simulink model "VIPR557StEnCtrl"  (R2018b)
settings: Solver=FixedStepDiscrete  StartTime=0.0  StopTime=10.0  FixedStep=0.01  RelTol=1e-3
undefined symbols (not defined in the file or in its folder): data, KeSMSw4SSecRwLtStLgrstUpwdDnwdOpenPos1_Val, PassStBkReclnEn_Clear, PassStBkReclnEn_Set, PassStFwdBkwdEn_Clear, PassStFwdBkwdEn_Set, SecRwRtStBkReclnEn_Clear, SecRwRtStBkReclnEn_Set, SecRwRtStFwdBkwdEn_Clear, SecRwRtStFwdBkwdEn_Set, SecRwRtStLgrstInwdOtwdEn_Clear, SecRwRtStLgrstInwdOtwdEn_Set, SecRwRtStLgrstUpwdDnwdEn_Clear, SecRwRtStLgrstUpwdDnwdEn_Set, ThdRwLtStBkReclnEn_Clear, ThdRwLtStBkReclnEn_Set, ThdRwLtStFwdBkwdEn_Clear, ThdRwLtStFwdBkwdEn_Set, ThdRwRtStBkReclnEn_Clear, ThdRwRtStBkReclnEn_Set, ThdRwRtStFwdBkwdEn_Clear, ThdRwRtStFwdBkwdEn_Set, ZeroREn_Clear, ZeroREn_Set
libraries: simulink x1
settings Model: Creator=sn2xws  LastModifiedBy=sn2xws
settings Model: ModifiedHistory=|
  | 2024.7.3 V3.0.0 557模式流程V1.9
  | 2024.8.16 V3.0.1  目标位置改为立即读取
  | 2024.8.22 V3.0.2 增加FirstTrig参数，智享目标位置计算改为只计算一次
  | 2024.8.30 V3.0.3 修复第一次无法调用问题
  | 2024.10.28 V3.0.4 6s版本不动三左
  | 2024.11.5 V3.0.5 6s版本不动三左更改逻辑错误，stateflow改为！7s
  | 2024.12.11 v3.0.6 CR953605
  | 2025.03.28 V3.0.7 CR1010402
  | 2025.04.07 V3.0.8 CR1010402 靠背位置无效。前后靠背电机都不动
  | 2025.6.25 V3.13.0 bug1068643 腿托流程偶发提前问题修复
  | 25.7.31 V3.13.1 CR 1100249
  | 25.9.12 V3.16.0 优化副驾占座后的动作（不恢复动作）
settings DataIOCC: SaveFormat=StructureWithTime
settings OptimizationCC: DefaultParameterBehavior=Inlined  EnhancedBackFolding=on  PassReuseOutputArgsAs=Individual arguments  ZeroExternalMemoryAtStartup=off  ZeroInternalMemoryAtStartup=off  OptimizeBlockOrder=speed  DifferentSizesBufferReuse=on  OptimizationCustomize=off
settings DebuggingCC: ParameterTunabilityLossMsg=error
settings SFSimCC: MATLABDynamicMemAlloc=off
settings RTWCC: SystemTargetFile=autosar.tlc  GenCodeOnly=on  TemplateMakefile=ert_default_tmf  Description=AUTOSAR  GenerateReport=on  IncludeHyperlinkInReport=on  LaunchReport=on  GenerateTraceInfo=on  GenerateTraceReport=on  GenerateTraceReportSl=on  GenerateTraceReportSf=on  GenerateTraceReportEml=on
settings CodeAppCC: ForceParamTrailComments=on  IgnoreCustomStorageClasses=off  OperatorAnnotations=on  SimulinkDataObjDesc=on  SFDataObjDesc=on  InsertBlockDesc=on
settings STFCustomTargetCC: TargetLangStandard=C99 (ISO)  MultiwordLength=256  ParMdlRefBuildCompliant=on  CompOptLevelCompliant=on  IncludeMdlTerminateFcn=off  CombineOutputUpdateFcns=on  SuppressErrorStatus=on  ERTCustomFileBanners=on  SupportNonFinite=off  SupportComplex=off  SupportContinuousTime=off  SupportNonInlinedSFcns=off  RemoveResetFunc=on  MATLABClassNameForMDSCustomization=Simulink.SoftwareTarget.ERTCustomization  AutosarCompliant=on  UseToolchainInfoCompliant=on  LookupTableObjectStructAxisOrder=2,1,3,4,...  LUTObjectStructOrderEvenSpacing=Size,Table,Breakpoints  SystemTargetFile=autosar.tlc
settings ERTTargetCC: TargetLangStandard=C99 (ISO)  ConcurrentExecutionCompliant=off  IncludeMdlTerminateFcn=off  SuppressErrorStatus=on  SupportNonFinite=off  SupportComplex=off  ModelStepFunctionPrototypeControlCompliant=off  CPPClassGenCompliant=off  AutosarCompliant=on  LookupTableObjectStructAxisOrder=2,1,3,4,...  LUTObjectStructOrderEvenSpacing=Size,Table,Breakpoints  InlinedParameterPlacement=NonHierarchical  ERTCustomFileTemplate=example_file_process.tlc  ERTFilePackagingFormat=Compact

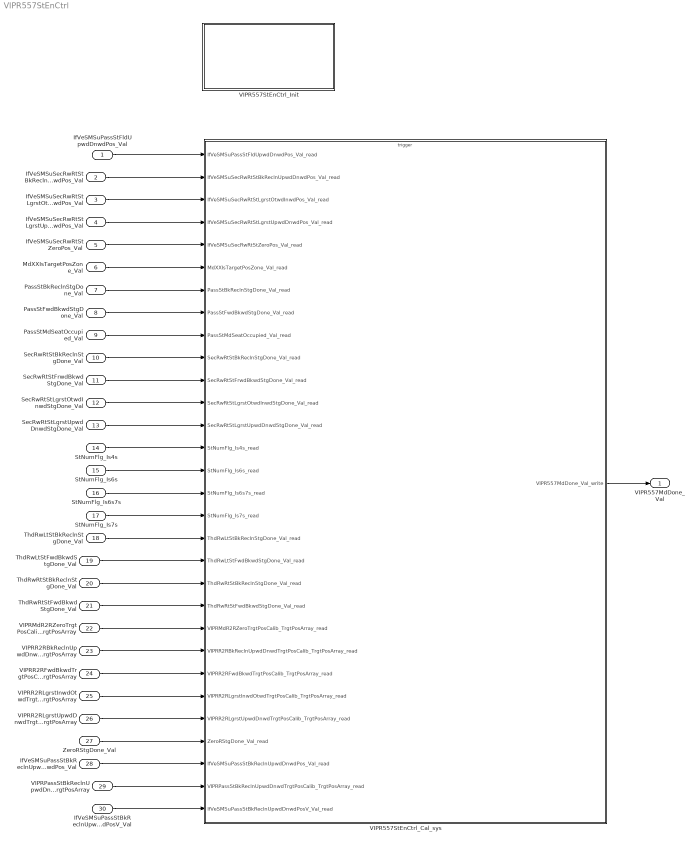
== system VIPR557StEnCtrl ==
  IfVeSMSuPassStFldUpwdDnwdPos_Val : Inport  OutDataTypeStr=uint16  PortDimensions=1
  IfVeSMSuSecRwRtStBkReclnUpwdDnwdPos_Val : Inport  Port=2  OutDataTypeStr=uint16  PortDimensions=1
  IfVeSMSuSecRwRtStLgrstOtwdInwdPos_Val : Inport  Port=3  OutDataTypeStr=uint16  PortDimensions=1
  IfVeSMSuSecRwRtStLgrstUpwdDnwdPos_Val : Inport  Port=4  OutDataTypeStr=uint16  PortDimensions=1
  IfVeSMSuSecRwRtStZeroPos_Val : Inport  Port=5  OutDataTypeStr=uint16  PortDimensions=1
  MdXXIsTargetPosZone_Val : Inport  Port=6  OutDataTypeStr=uint32  PortDimensions=1
  PassStBkReclnStgDone_Val : Inport  Port=7  OutDataTypeStr=boolean  PortDimensions=1
  PassStFwdBkwdStgDone_Val : Inport  Port=8  OutDataTypeStr=boolean  PortDimensions=1
  PassStMdSeatOccupied_Val : Inport  Port=9  OutDataTypeStr=boolean  PortDimensions=1
  SecRwRtStBkReclnStgDone_Val : Inport  Port=10  OutDataTypeStr=boolean  PortDimensions=1
  SecRwRtStFrwdBkwdStgDone_Val : Inport  Port=11  OutDataTypeStr=boolean  PortDimensions=1
  SecRwRtStLgrstOtwdInwdStgDone_Val : Inport  Port=12  OutDataTypeStr=boolean  PortDimensions=1
  SecRwRtStLgrstUpwdDnwdStgDone_Val : Inport  Port=13  OutDataTypeStr=boolean  PortDimensions=1
  StNumFlg_Is4s : Inport  Port=14  OutDataTypeStr=boolean  PortDimensions=1
  StNumFlg_Is6s : Inport  Port=15  OutDataTypeStr=boolean  PortDimensions=1
  StNumFlg_Is6s7s : Inport  Port=16  OutDataTypeStr=boolean  PortDimensions=1
  StNumFlg_Is7s : Inport  Port=17  OutDataTypeStr=boolean  PortDimensions=1
  ThdRwLtStBkReclnStgDone_Val : Inport  Port=18  OutDataTypeStr=boolean  PortDimensions=1
  ThdRwLtStFwdBkwdStgDone_Val : Inport  Port=19  OutDataTypeStr=boolean  PortDimensions=1
  ThdRwRtStBkReclnStgDone_Val : Inport  Port=20  OutDataTypeStr=boolean  PortDimensions=1
  ThdRwRtStFwdBkwdStgDone_Val : Inport  Port=21  OutDataTypeStr=boolean  PortDimensions=1
  VIPRMdR2RZeroTrgtPosCalib_TrgtPosArray : Inport  Description=|  Port=22  OutDataTypeStr=uint16  PortDimensions=3
      | 0:Pos
      | 1:Max
      | 2:Min
  VIPRR2RBkReclnUpwdDnwdTrgtPosCalib_TrgtPosArray : Inport  Description=|  Port=23  OutDataTypeStr=uint16  PortDimensions=3
      | 0:Pos
      | 1:Max
      | 2:Min
  VIPRR2RFwdBkwdTrgtPosCalib_TrgtPosArray : Inport  Description=|  Port=24  OutDataTypeStr=uint16  PortDimensions=3
      | 0:Pos
      | 1:Max
      | 2:Min
  VIPRR2RLgrstInwdOtwdTrgtPosCalib_TrgtPosArray : Inport  Description=|  Port=25  OutDataTypeStr=uint16  PortDimensions=3
      | 0:Pos
      | 1:Max
      | 2:Min
  VIPRR2RLgrstUpwdDnwdTrgtPosCalib_TrgtPosArray : Inport  Description=|  Port=26  OutDataTypeStr=uint16  PortDimensions=3
      | 0:Pos
      | 1:Max
      | 2:Min
  ZeroRStgDone_Val : Inport  Port=27  OutDataTypeStr=boolean  PortDimensions=1
  IfVeSMSuPassStBkReclnUpwdDnwdPos_Val : Inport  Port=28  OutDataTypeStr=uint16  PortDimensions=1
  VIPRPassStBkReclnUpwdDnwdTrgtPosCalib_TrgtPosArray : Inport  Description=|  Port=29  OutDataTypeStr=uint16  PortDimensions=3
      | 0:Pos
      | 1:Max
      | 2:Min
  IfVeSMSuPassStBkReclnUpwdDnwdPosV_Val : Inport  Port=30  OutDataTypeStr=boolean  PortDimensions=1
  VIPR557StEnCtrl_Cal_sys : Subsystem
  VIPR557StEnCtrl_Init : Subsystem
  VIPR557MdDone_Val : Outport  OutDataTypeStr=uint8  PortDimensions=1
  wires:
  IfVeSMSuPassStFldUpwdDnwdPos_Val/1 -> VIPR557StEnCtrl_Cal_sys/1(IfVeSMSuPassStFldUpwdDnwdPos_Val_read)
  IfVeSMSuSecRwRtStBkReclnUpwdDnwdPos_Val/1 -> VIPR557StEnCtrl_Cal_sys/2(IfVeSMSuSecRwRtStBkReclnUpwdDnwdPos_Val_read)
  IfVeSMSuSecRwRtStLgrstOtwdInwdPos_Val/1 -> VIPR557StEnCtrl_Cal_sys/3(IfVeSMSuSecRwRtStLgrstOtwdInwdPos_Val_read)
  IfVeSMSuSecRwRtStLgrstUpwdDnwdPos_Val/1 -> VIPR557StEnCtrl_Cal_sys/4(IfVeSMSuSecRwRtStLgrstUpwdDnwdPos_Val_read)
  IfVeSMSuSecRwRtStZeroPos_Val/1 -> VIPR557StEnCtrl_Cal_sys/5(IfVeSMSuSecRwRtStZeroPos_Val_read)
  MdXXIsTargetPosZone_Val/1 -> VIPR557StEnCtrl_Cal_sys/6(MdXXIsTargetPosZone_Val_read)
  PassStBkReclnStgDone_Val/1 -> VIPR557StEnCtrl_Cal_sys/7(PassStBkReclnStgDone_Val_read)
  PassStFwdBkwdStgDone_Val/1 -> VIPR557StEnCtrl_Cal_sys/8(PassStFwdBkwdStgDone_Val_read)
  PassStMdSeatOccupied_Val/1 -> VIPR557StEnCtrl_Cal_sys/9(PassStMdSeatOccupied_Val_read)
  SecRwRtStBkReclnStgDone_Val/1 -> VIPR557StEnCtrl_Cal_sys/10(SecRwRtStBkReclnStgDone_Val_read)
  SecRwRtStFrwdBkwdStgDone_Val/1 -> VIPR557StEnCtrl_Cal_sys/11(SecRwRtStFrwdBkwdStgDone_Val_read)
  SecRwRtStLgrstOtwdInwdStgDone_Val/1 -> VIPR557StEnCtrl_Cal_sys/12(SecRwRtStLgrstOtwdInwdStgDone_Val_read)
  SecRwRtStLgrstUpwdDnwdStgDone_Val/1 -> VIPR557StEnCtrl_Cal_sys/13(SecRwRtStLgrstUpwdDnwdStgDone_Val_read)
  StNumFlg_Is4s/1 -> VIPR557StEnCtrl_Cal_sys/14(StNumFlg_Is4s_read)
  StNumFlg_Is6s/1 -> VIPR557StEnCtrl_Cal_sys/15(StNumFlg_Is6s_read)
  StNumFlg_Is6s7s/1 -> VIPR557StEnCtrl_Cal_sys/16(StNumFlg_Is6s7s_read)
  StNumFlg_Is7s/1 -> VIPR557StEnCtrl_Cal_sys/17(StNumFlg_Is7s_read)
  ThdRwLtStBkReclnStgDone_Val/1 -> VIPR557StEnCtrl_Cal_sys/18(ThdRwLtStBkReclnStgDone_Val_read)
  ThdRwLtStFwdBkwdStgDone_Val/1 -> VIPR557StEnCtrl_Cal_sys/19(ThdRwLtStFwdBkwdStgDone_Val_read)
  ThdRwRtStBkReclnStgDone_Val/1 -> VIPR557StEnCtrl_Cal_sys/20(ThdRwRtStBkReclnStgDone_Val_read)
  ThdRwRtStFwdBkwdStgDone_Val/1 -> VIPR557StEnCtrl_Cal_sys/21(ThdRwRtStFwdBkwdStgDone_Val_read)
  VIPRMdR2RZeroTrgtPosCalib_TrgtPosArray/1 -> VIPR557StEnCtrl_Cal_sys/22(VIPRMdR2RZeroTrgtPosCalib_TrgtPosArray_read)
  VIPRR2RBkReclnUpwdDnwdTrgtPosCalib_TrgtPosArray/1 -> VIPR557StEnCtrl_Cal_sys/23(VIPRR2RBkReclnUpwdDnwdTrgtPosCalib_TrgtPosArray_read)
  VIPRR2RFwdBkwdTrgtPosCalib_TrgtPosArray/1 -> VIPR557StEnCtrl_Cal_sys/24(VIPRR2RFwdBkwdTrgtPosCalib_TrgtPosArray_read)
  VIPRR2RLgrstInwdOtwdTrgtPosCalib_TrgtPosArray/1 -> VIPR557StEnCtrl_Cal_sys/25(VIPRR2RLgrstInwdOtwdTrgtPosCalib_TrgtPosArray_read)
  VIPRR2RLgrstUpwdDnwdTrgtPosCalib_TrgtPosArray/1 -> VIPR557StEnCtrl_Cal_sys/26(VIPRR2RLgrstUpwdDnwdTrgtPosCalib_TrgtPosArray_read)
  ZeroRStgDone_Val/1 -> VIPR557StEnCtrl_Cal_sys/27(ZeroRStgDone_Val_read)
  VIPR557StEnCtrl_Cal_sys/1(VIPR557MdDone_Val_write) -> VIPR557MdDone_Val/1
  IfVeSMSuPassStBkReclnUpwdDnwdPos_Val/1 -> VIPR557StEnCtrl_Cal_sys/28(IfVeSMSuPassStBkReclnUpwdDnwdPos_Val_read)
  VIPRPassStBkReclnUpwdDnwdTrgtPosCalib_TrgtPosArray/1 -> VIPR557StEnCtrl_Cal_sys/29(VIPRPassStBkReclnUpwdDnwdTrgtPosCalib_TrgtPosArray_read)
  IfVeSMSuPassStBkReclnUpwdDnwdPosV_Val/1 -> VIPR557StEnCtrl_Cal_sys/30(IfVeSMSuPassStBkReclnUpwdDnwdPosV_Val_read)

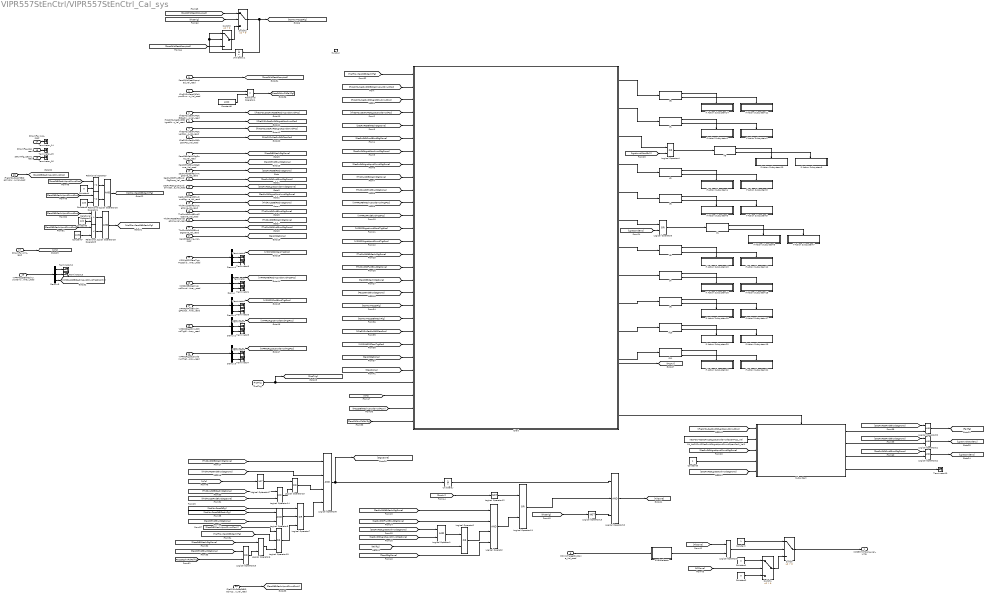
== system VIPR557StEnCtrl/VIPR557StEnCtrl_Cal_sys ==
  IfVeSMSuPassStFldUpwdDnwdPos_Val_read : Inport
  IfVeSMSuSecRwRtStBkReclnUpwdDnwdPos_Val_read : Inport  Port=2
  IfVeSMSuSecRwRtStLgrstOtwdInwdPos_Val_read : Inport  Port=3
  IfVeSMSuSecRwRtStLgrstUpwdDnwdPos_Val_read : Inport  Port=4
  IfVeSMSuSecRwRtStZeroPos_Val_read : Inport  Port=5
  MdXXIsTargetPosZone_Val_read : Inport  Port=6
  PassStBkReclnStgDone_Val_read : Inport  Port=7
  PassStFwdBkwdStgDone_Val_read : Inport  Port=8
  PassStMdSeatOccupied_Val_read : Inport  Port=9
  SecRwRtStBkReclnStgDone_Val_read : Inport  Port=10
  SecRwRtStFrwdBkwdStgDone_Val_read : Inport  Port=11
  SecRwRtStLgrstOtwdInwdStgDone_Val_read : Inport  Port=12
  SecRwRtStLgrstUpwdDnwdStgDone_Val_read : Inport  Port=13
  StNumFlg_Is4s_read : Inport  Port=14
  StNumFlg_Is6s_read : Inport  Port=15
  StNumFlg_Is6s7s_read : Inport  Port=16
  StNumFlg_Is7s_read : Inport  Port=17
  ThdRwLtStBkReclnStgDone_Val_read : Inport  Port=18
  ThdRwLtStFwdBkwdStgDone_Val_read : Inport  Port=19
  ThdRwRtStBkReclnStgDone_Val_read : Inport  Port=20
  ThdRwRtStFwdBkwdStgDone_Val_read : Inport  Port=21
  VIPRMdR2RZeroTrgtPosCalib_TrgtPosArray_read : Inport  Port=22
  VIPRR2RBkReclnUpwdDnwdTrgtPosCalib_TrgtPosArray_read : Inport  Port=23
  VIPRR2RFwdBkwdTrgtPosCalib_TrgtPosArray_read : Inport  Port=24
  VIPRR2RLgrstInwdOtwdTrgtPosCalib_TrgtPosArray_read : Inport  Port=25
  VIPRR2RLgrstUpwdDnwdTrgtPosCalib_TrgtPosArray_read : Inport  Port=26
  ZeroRStgDone_Val_read : Inport  Port=27
  IfVeSMSuPassStBkReclnUpwdDnwdPos_Val_read : Inport  Port=28
  VIPRPassStBkReclnUpwdDnwdTrgtPosCalib_TrgtPosArray_read : Inport  Port=29
  IfVeSMSuPassStBkReclnUpwdDnwdPosV_Val_read : Inport  Port=30
  function : TriggerPort  TriggerType=function-call  IsSimulinkFunction=on  FunctionName=VIPR557StEnCtrl_Cal  VariantControl=(inherit)
  32BitSelector : Subsystem  mask(32 Bit Selector){BitNum=11}
      mask prompts: BitNum "Select Bit Number"
      mask help: Allows selection of a particular bit (0-31) out of a packed word up to 32 bits long. Output will be true if the bit number selected via the mask parameter is equal to one.
      mask TypeOptions BitNum: 0 | 1 | 2 | 3 | 4 | 5 | 6 | 7 | 8 | 9 | 10 | 11 | 12 | 13 | 14 | 15 | 16 | 17 | 18 | 19 | 20 | 21 | 22 | 23 | 24 | 25 | 26 | 27 | 28 | 29 | 30 | 31
      mask Display:
      | text(0.5, 0.8,'BIT','horizontalAlignment','center')
      | text(0.5, 0.5,'SELECTOR','horizontalAlignment','center')
      | text(0.5, 0.2,['-- Bit ',char(get_param(gcb,'BitNum')),' --'],'horizontalAlignment','center')
  Chart : Stateflow chart  TreatAsAtomicUnit=on
  Constant : Constant  OutDataTypeStr=uint8
  Constant1 : Constant  Value=2  OutDataTypeStr=uint8
  Constant2 : Constant  Value=0  OutDataTypeStr=uint8
  Constant3 : Constant  OutDataTypeStr=boolean
  Constant4 : Constant  Value=0  OutDataTypeStr=uint16
  Constant5 : Constant  Value=120  OutDataTypeStr=uint16
  Constant6 : Constant  Value=120  OutDataTypeStr=uint16
  Constant7 : Constant  Value=1692  OutDataTypeStr=uint16
  Constant8 : Constant  Value=4000  OutDataTypeStr=uint16
  Demux{,1..5} (6 alike) : Demux  Outputs=3
  If Action Subsystem1 : Subsystem  TreatAsAtomicUnit=on
  If Action Subsystem10 : Subsystem  TreatAsAtomicUnit=on
  If Action Subsystem11 : Subsystem  TreatAsAtomicUnit=on
  If Action Subsystem12 : Subsystem  TreatAsAtomicUnit=on
  If Action Subsystem13 : Subsystem  TreatAsAtomicUnit=on
  If Action Subsystem14 : Subsystem  TreatAsAtomicUnit=on
  If Action Subsystem15 : Subsystem  TreatAsAtomicUnit=on
  If Action Subsystem16 : Subsystem  TreatAsAtomicUnit=on
  If Action Subsystem17 : Subsystem  TreatAsAtomicUnit=on
  If Action Subsystem18 : Subsystem  TreatAsAtomicUnit=on
  If Action Subsystem19 : Subsystem  TreatAsAtomicUnit=on
  If Action Subsystem2 : Subsystem  TreatAsAtomicUnit=on
  If Action Subsystem20 : Subsystem  TreatAsAtomicUnit=on
  If Action Subsystem21 : Subsystem  TreatAsAtomicUnit=on
  If Action Subsystem22 : Subsystem  TreatAsAtomicUnit=on
  If Action Subsystem3 : Subsystem  TreatAsAtomicUnit=on
  If Action Subsystem4 : Subsystem  TreatAsAtomicUnit=on
  If Action Subsystem5 : Subsystem  TreatAsAtomicUnit=on
  If Action Subsystem6 : Subsystem  TreatAsAtomicUnit=on
  If Action Subsystem7 : Subsystem  TreatAsAtomicUnit=on
  If Action Subsystem8 : Subsystem  TreatAsAtomicUnit=on
  If Action Subsystem9 : Subsystem  TreatAsAtomicUnit=on
  If{1..11} (11 alike) : If  IfExpression=u1
  Logical Operator : Logic  Inputs=4  AllPortsSameDT=off  OutDataTypeStr=boolean
  Logical Operator{1,5..6,9,14,16,18,20..22} (10 alike) : Logic  AllPortsSameDT=off  OutDataTypeStr=boolean
  Logical Operator10 : Logic  Inputs=3  AllPortsSameDT=off  OutDataTypeStr=boolean
  Logical Operator{2..4,11,15,23} (6 alike) : Logic  Operator=OR  AllPortsSameDT=off  OutDataTypeStr=boolean
  Logical Operator12 : Logic  Operator=NOT  AllPortsSameDT=off  OutDataTypeStr=boolean
  Logical Operator13 : Logic  Operator=NOT  AllPortsSameDT=off  OutDataTypeStr=boolean
  Logical Operator17 : Logic  Operator=NOT  Inputs=1  AllPortsSameDT=off  OutDataTypeStr=boolean
  Logical Operator19 : Logic  Operator=OR  Inputs=3  AllPortsSameDT=off  OutDataTypeStr=boolean
  Logical Operator7 : Logic  Operator=OR  Inputs=3  AllPortsSameDT=off  OutDataTypeStr=boolean
  Logical Operator8 : Logic  Inputs=4  AllPortsSameDT=off  OutDataTypeStr=boolean
  PA_KeSMSw4SSecRwLtStLgrstUpwdDnwdOpenPos1_Val1 : Constant  Value=KeSMSw4SSecRwLtStLgrstUpwdDnwdOpenPos1_Val
  Relational Operator : RelationalOperator  OutDataTypeStr=boolean  RndMeth=Simplest
  Relational Operator1 : RelationalOperator  Operator=<=  OutDataTypeStr=boolean  RndMeth=Simplest
  Relational Operator2 : RelationalOperator  Operator=>  OutDataTypeStr=boolean  RndMeth=Simplest
  Relational Operator3 : RelationalOperator  Operator=<  OutDataTypeStr=boolean  RndMeth=Simplest
  Relational Operator4 : RelationalOperator  Operator=<  OutDataTypeStr=boolean  RndMeth=Simplest
  Subsystem : Subsystem
  Switch{,1..3} (4 alike) : Switch  Criteria=u2 > Threshold
  Terminator{,1..10,12..13} (13 alike) : Terminator
  Terminator_14 : Terminator
  Terminator_15 : Terminator
  Terminator_16 : Terminator
  Unit Delay : UnitDelay  SampleTime=-1
  Unit Delay1 : UnitDelay  SampleTime=-1
  FirstTrig : ArgIn  OutDataTypeStr=boolean  ArgumentName=FirstTrig
  VIPR557MdDone_Val_write : Outport
      settings: EnsureOutportIsVirtual=on
  wires:
  StNumFlg_Is4s_read/1 -> Terminator_14/1
  StNumFlg_Is6s_read/1 -> Terminator_15/1
  StNumFlg_Is6s7s_read/1 -> Terminator_16/1
  StNumFlg_Is7s_read/1 -> [Is7s]
  ThdRwRtStBkReclnStgDone_Val_read/1 -> [ThdRwRtStBkReclnStgDone]
  IfVeSMSuSecRwRtStBkReclnUpwdDnwdPos_Val_read/1 -> [IfVeSMSuSecRwRtStBkReclnUpwdDnwdPos]
  ThdRwRtStFwdBkwdStgDone_Val_read/1 -> [ThdRwRtStFwdBkwdStgDone]
  ThdRwLtStFwdBkwdStgDone_Val_read/1 -> [ThdRwLtStFwdBkwdStgDone]
  PassStBkReclnStgDone_Val_read/1 -> [PassStBkReclnStgDone]
  SecRwRtStLgrstOtwdInwdStgDone_Val_read/1 -> [SecRwRtStLgrstOtwdInwdStgDone]
  PassStFwdBkwdStgDone_Val_read/1 -> [PassStFwdBkwdStgDone]
  SecRwRtStLgrstUpwdDnwdStgDone_Val_read/1 -> [SecRwRtStLgrstUpwdDnwdStgDone]
  IfVeSMSuSecRwRtStLgrstOtwdInwdPos_Val_read/1 -> [IfVeSMSuSecRwRtStLgrstOtwdInwdPos]
  IfVeSMSuSecRwRtStLgrstUpwdDnwdPos_Val_read/1 -> [IfVeSMSuSecRwRtStLgrstUpwdDnwdPos]
  SecRwRtStFrwdBkwdStgDone_Val_read/1 -> [SecRwRtStFrwdBkwdStgDone]
  SecRwRtStBkReclnStgDone_Val_read/1 -> [SecRwRtStBkReclnStgDone]
  ThdRwLtStBkReclnStgDone_Val_read/1 -> [ThdRwLtStBkReclnStgDone]
  Demux/2 -> Terminator/1
  Demux2/3 -> Terminator5/1
  Demux1/1 -> [VIPRR2RFwdBkwdTrgtPos]
  Demux3/3 -> Terminator7/1
  VIPRR2RLgrstInwdOtwdTrgtPosCalib_TrgtPosArray_read/1 -> Demux2/1
  Demux2/2 -> Terminator4/1
  Demux3/1 -> [VIPRR2RLgrstUpwdDnwdTrgtPos]
  Demux/3 -> Terminator1/1
  VIPRR2RFwdBkwdTrgtPosCalib_TrgtPosArray_read/1 -> Demux1/1
  Demux2/1 -> [VIPRR2RLgrstInwdOtwdTrgtPos]
  Demux1/3 -> Terminator3/1
  Demux/1 -> [VIPRR2RBkReclnUpwdDnwdTrgtPos]
  VIPRR2RLgrstUpwdDnwdTrgtPosCalib_TrgtPosArray_read/1 -> Demux3/1
  VIPRR2RBkReclnUpwdDnwdTrgtPosCalib_TrgtPosArray_read/1 -> Demux/1
  Demux3/2 -> Terminator6/1
  Demux1/2 -> Terminator2/1
  VIPRMdR2RZeroTrgtPosCalib_TrgtPosArray_read/1 -> Demux4/1
  Demux4/1 -> [VIPRMdR2RZeroTrgtPos]
  Demux4/3 -> Terminator9/1
  Demux4/2 -> Terminator8/1
  ZeroRStgDone_Val_read/1 -> [ZeroRStgDone]
  IfVeSMSuSecRwRtStZeroPos_Val_read/1 -> [IfVeSMSuSecRwRtStZeroPos]
  Chart/2(SecRwLtStFrwdBkwdEn) -> If1/1
  [VIPRR2RLgrstUpwdDnwdTrgtPos] -> Chart/14(VIPLR2LLgrstUpwdDnwdTrgtPos)
  [SecRwRtStLgrstUpwdDnwdStgDone] -> Logical Operator1/2
  [IfVeSMSuSecRwRtStLgrstOtwdInwdPos] -> Chart/3(IfVeSMSuSecRwLtStLgrstOtwdInwdPos)
  [SecRwRtStFrwdBkwdStgDone] -> Chart/6(SecRwLtStFrwdBkwdStgDone)
  [SecRwRtStLgrstUpwdDnwdStgDone] -> Chart/8(SecRwLtStLgrstUpwdDnwdStgDone)
  If3/1 -> If Action Subsystem6/Action
  [SecRwRtStLgrstOtwdInwdStgDone] -> Logical Operator1/1
  If4/1 -> If Action Subsystem8/Action
  If1/1 -> If Action Subsystem2/Action
  Chart/3(SecRwLtStLgrstOtwdInwdEn) -> Logical Operator4/1
  If8/2 -> If Action Subsystem11/Action
  Subsystem/4(FtrstEn) -> Terminator10/1
  Chart/4(ThdRwLtStBkReclnEn) -> If2/1
  [LgrstInwdOtwdEn2] -> Logical Operator4/2
  If4/2 -> If Action Subsystem7/Action
  If2/2 -> If Action Subsystem3/Action
  [VIPRR2RBkReclnUpwdDnwdTrgtPos] -> Chart/11(VIPLR2LBkReclnUpwdDnwdTrgtPos)
  If3/2 -> If Action Subsystem5/Action
  [IfVeSMSuSecRwRtStLgrstUpwdDnwdPos] -> Subsystem/1(LgrstUpwdDnwdPos)
  Chart/6(SecRwLtStLgrstUpwdDnwdEn) -> Logical Operator3/1
  [NotMovPassStBkReclnFlg] -> Logical Operator5/1
  Chart/10(PassStFwdBkwdEn) -> If10/1
  [NotMovPassStBkReclnFlg] -> Chart/20(NotMovPassStBkReclnFlg)
  If6/1 -> If Action Subsystem13/Action
  [SecRwRtStLgrstOtwdInwdStgDone] -> Chart/7(SecRwLtStLgrstOtwdInwdStgDone)
  [PassStBkReclnStgDone] -> Chart/17(PassStBkReclnStgDone)
  [ThdRwLtStFwdBkwdStgDone] -> Chart/10(ThdRwLtStFwdBkwdStgDone)
  If9/2 -> If Action Subsystem17/Action
  Constant3/1 -> Subsystem/4(FtrstStgDone)
  If9/1 -> If Action Subsystem18/Action
  If7/2 -> If Action Subsystem15/Action
  Chart/13(LgrstOpn()) -> Subsystem/Trigger
  [VIPRR2RLgrstInwdOtwdTrgtPos] -> Chart/13(VIPLR2LLgrstInwdOtwdTrgtPos)
  [IfVeSMSuSecRwRtStLgrstUpwdDnwdPos] -> Chart/4(IfVeSMSuSecRwLtStLgrstUpwdDnwdPos)
  If6/2 -> If Action Subsystem12/Action
  Logical Operator5/1 -> Logical Operator7/2
  Chart/7(ThdRwRtStBkReclnEn) -> If6/1
  [NotMovPassStFlg] -> Chart/19(NotMovPassStFlg)
  If5/2 -> If Action Subsystem9/Action
  Chart/8(ThdRwRtStFwdBkwdEn) -> If7/1
  If10/2 -> If Action Subsystem19/Action
  [SecRwRtStLgrstOtwdInwdStgDone] -> Subsystem/5(LgrstInwdStgDone)
  Logical Operator4/1 -> If5/1
  [Failflg] -> Logical Operator2/2
  If5/1 -> If Action Subsystem10/Action
  [PassStBkReclnStgDone] -> Logical Operator6/1
  If10/1 -> If Action Subsystem20/Action
  [PassStFwdBkwdStgDone] -> Chart/18(PassStFwdBkwdStgDone)
  Chart/5(ThdRwLtStFwdBkwdEn) -> If3/1
  [SecRwRtStLgrstUpwdDnwdStgDone] -> Subsystem/3(LgrstUpwdStgDone)
  If8/1 -> If Action Subsystem14/Action
  [ThdRwRtStBkReclnStgDone] -> Chart/15(ThdRwRtStBkReclnStgDone)
  Logical Operator1/1 -> Logical Operator2/1
  Chart/9(PassStBkReclnEn) -> If9/1
  If1/2 -> If Action Subsystem1/Action
  If7/1 -> If Action Subsystem16/Action
  [NotMovPassStFlg] -> Logical Operator7/1
  [ThdRwRtStFwdBkwdStgDone] -> Chart/16(ThdRwRtStFwdBkwdStgDone)
  PA_KeSMSw4SSecRwLtStLgrstUpwdDnwdOpenPos1_Val1/1 -> Subsystem/2(LgrstUpwdDnwdOpenPos1)
  [IfVeSMSuSecRwRtStBkReclnUpwdDnwdPos] -> Chart/2(IfVeSMSuSecRwLtStBkReclnUpwdDnwdPos)
  [LgrstUpwdEn2] -> Logical Operator3/2
  Chart/1(SecRwLtStBkReclnEn) -> If8/1
  [ThdRwLtStBkReclnStgDone] -> Chart/9(ThdRwLtStBkReclnStgDone)
  Logical Operator3/1 -> If4/1
  [SecRwRtStBkReclnStgDone] -> Chart/5(SecRwLtStBkReclnStgDone)
  If2/1 -> If Action Subsystem4/Action
  [VIPRR2RFwdBkwdTrgtPos] -> Chart/12(VIPLR2LFwdBkwdTrgtPos)
  Constant2/1 -> Switch1/3
  Switch1/1 -> Switch/3
  MdXXIsTargetPosZone_Val_read/1 -> 32BitSelector/1(x)
  Constant1/1 -> Switch1/1
  [AllDone] -> Switch1/2
  Switch/1 -> VIPR557MdDone_Val_write/1
  Constant/1 -> Switch/1
  Logical Operator9/1 -> Switch/2
  32BitSelector/1(y) -> Logical Operator9/2
  [AllDone] -> Logical Operator9/1
  [ThdRwRtStBkReclnStgDone] -> Logical Operator8/1
  [ThdRwRtStFwdBkwdStgDone] -> Logical Operator8/2
  Logical Operator7/1 -> Logical Operator8/4
  Logical Operator8/1 -> [Stg1Done], Unit Delay/1
  [IfVeSMSuSecRwRtStZeroPos] -> Chart/21(IfVeSMSuSecRwRtStZeroPos)
  [VIPRMdR2RZeroTrgtPos] -> Chart/22(VIPRMdR2RZeroTrgtPos)
  [ZeroRStgDone] -> Chart/23(ZeroRStgDone)
  [Stg1Done] -> Chart/24(Stg1Done)
  If11/1 -> If Action Subsystem22/Action
  If11/2 -> If Action Subsystem21/Action
  Chart/11(SecRwStZeroEn) -> If11/1
  Chart/12(PosAvl) -> [PosAvl]
  [SecRwRtStBkReclnStgDone] -> Logical Operator/1
  [SecRwRtStFrwdBkwdStgDone] -> Logical Operator/2
  Logical Operator2/1 -> Logical Operator/3
  [ZeroRStgDone] -> Logical Operator/4
  Logical Operator10/1 -> [AllDone]
  Logical Operator11/1 -> Logical Operator10/2
  [PosAvl] -> Logical Operator12/1
  Logical Operator12/1 -> Logical Operator11/1
  Logical Operator/1 -> Logical Operator11/2
  Unit Delay/1 -> Logical Operator10/1
  PassStMdSeatOccupied_Val_read/1 -> [PassStMdSeatOccupied]
  FirstTrig/1 -> Chart/25(FirstTrig), [FirstTrig]
  Logical Operator13/1 -> Logical Operator10/3
  [FirstTrig] -> Logical Operator13/1
  [Is7s] -> Chart/26(is7s)
  [ThdRwLtStFwdBkwdStgDone] -> Logical Operator14/2
  [ThdRwLtStBkReclnStgDone] -> Logical Operator14/1
  Logical Operator15/1 -> Logical Operator8/3
  Logical Operator14/1 -> Logical Operator15/2
  [Is7s] -> Logical Operator17/1
  Logical Operator17/1 -> Logical Operator15/1
  VIPRPassStBkReclnUpwdDnwdTrgtPosCalib_TrgtPosArray_read/1 -> Demux5/1
  Constant4/1 -> Relational Operator/2
  Relational Operator/1 -> Logical Operator16/1
  Relational Operator1/1 -> Logical Operator16/2
  Constant5/1 -> Relational Operator1/2
  Logical Operator16/1 -> [NotMovPassStBkReclnFlg]
  IfVeSMSuPassStBkReclnUpwdDnwdPos_Val_read/1 -> [PassStBkReclnUpwdDnwdPos]
  [PassStBkReclnUpwdDnwdPos] -> Relational Operator/1
  [PassStBkReclnUpwdDnwdPos] -> Relational Operator1/1
  Constant7/1 -> Relational Operator3/2
  [PassStBkReclnUpwdDnwdPos] -> Relational Operator2/1
  Relational Operator3/1 -> Logical Operator18/2
  Relational Operator2/1 -> Logical Operator18/1
  Constant6/1 -> Relational Operator2/2
  [PassStBkReclnUpwdDnwdPos] -> Relational Operator3/1
  Logical Operator18/1 -> [HalfMovPassStBkReclnFlg]
  [HalfMovPassStBkReclnFlg] -> Chart/1(HalfMovPassStBkReclnFlg)
  IfVeSMSuPassStFldUpwdDnwdPos_Val_read/1 -> Relational Operator4/1
  Demux5/1 -> Terminator12/1
  Demux5/2 -> Terminator13/1
  Demux5/3 -> [VIPRPassStBkReclnUpwdDnwdTrgtPosMin]
  [PassStFwdBkwdStgDone] -> Logical Operator5/2
  [HalfMovPassStBkReclnFlg] -> Logical Operator19/2
  Logical Operator19/1 -> Logical Operator7/3
  Logical Operator6/1 -> Logical Operator19/3
  IfVeSMSuPassStBkReclnUpwdDnwdPosV_Val_read/1 -> [PassStBkReclnUpwdDnwdPosV]
  [PassStBkReclnUpwdDnwdPosV] -> Chart/27(IfVeSMSuPassStBkReclnUpwdDnwdPosV)
  [PassStBkReclnUpwdDnwdPosV] -> Logical Operator19/1
  [SecRwRtStFrwdBkwdStgDone] -> Logical Operator20/1
  Logical Operator20/1 -> [Failflg]
  Subsystem/1(Failflg) -> Logical Operator20/2
  Logical Operator21/1 -> [LgrstInwdOtwdEn2]
  Logical Operator22/1 -> [LgrstUpwdEn2]
  [SecRwRtStFrwdBkwdStgDone] -> Logical Operator21/1
  [SecRwRtStFrwdBkwdStgDone] -> Logical Operator22/1
  Subsystem/2(LgrstInwdOtwdEn) -> Logical Operator21/2
  Subsystem/3(LgrstUpwdDnwdEn) -> Logical Operator22/2
  Logical Operator23/1 -> Logical Operator6/2
  [PassStFwdBkwdStgDone] -> Logical Operator23/1
  [PassStCshnFldFailflg] -> Logical Operator23/2
  [PassStCshnFldFailflg] -> Chart/28(PassStCshnFldFailflg)
  Relational Operator4/1 -> [PassStCshnFldFailflg]
  Constant8/1 -> Relational Operator4/2
  [FirstTrig] -> Switch2/2
  [PassStMdSeatOccupied] -> Switch2/1
  Switch2/1 -> Unit Delay1/1, [NotMovPassStFlg]
  Unit Delay1/1 -> Switch3/1, Switch3/2
  [PassStMdSeatOccupied] -> Switch3/3
  Switch3/1 -> Switch2/3

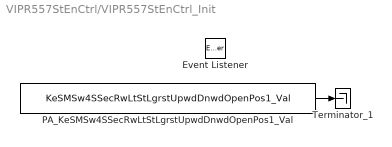
== system VIPR557StEnCtrl/VIPR557StEnCtrl_Init ==
  Event Listener : EventListener  EventName=reset
  PA_KeSMSw4SSecRwLtStLgrstUpwdDnwdOpenPos1_Val : Constant  Value=KeSMSw4SSecRwLtStLgrstUpwdDnwdOpenPos1_Val
  Terminator_1 : Terminator
  wires:
  PA_KeSMSw4SSecRwLtStLgrstUpwdDnwdOpenPos1_Val/1 -> Terminator_1/1

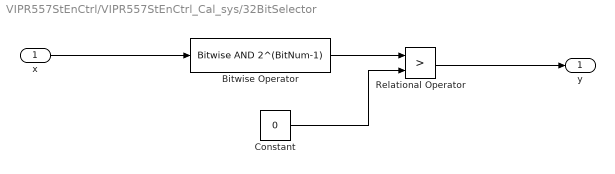
== system VIPR557StEnCtrl/VIPR557StEnCtrl_Cal_sys/32BitSelector ==
  x : Inport
  Bitwise Operator : simulink/Logic and Bit Operations/Bitwise Operator  logicop=AND  UseBitMask=on  BitMask=2^(BitNum-1)  BitMaskRealWorld=Stored Integer
  Constant : Constant  Value=0  OutDataTypeStr=uint32
  Relational Operator : RelationalOperator  Operator=>  OutDataTypeStr=boolean  RndMeth=Simplest
  y : Outport
  wires:
  Relational Operator/1 -> y/1
  Constant/1 -> Relational Operator/2
  x/1 -> Bitwise Operator/1
  Bitwise Operator/1 -> Relational Operator/1

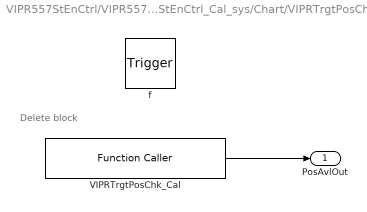
== system VIPR557StEnCtrl/VIPR557StEnCtrl_Cal_sys/Chart/VIPRTrgtPosChk ==
  note: Delete block
  f : TriggerPort  TriggerType=function-call  VariantControl=(inherit)
      settings: CopyFcn=Stateflow.SLINSF.SimulinkMan.removeBlockPreDeleteFcn  PreDeleteFcn=Stateflow.SLINSF.SimulinkMan.unsafePredeleteFcn
  VIPRTrgtPosChk_Cal : FunctionCaller  FunctionPrototype=PosAvl = VIPRTrgtPosChk_Cal()  OutputArgumentSpecifications=uint8(1)
  PosAvlOut : Outport
  wires:
  VIPRTrgtPosChk_Cal/1 -> PosAvlOut/1

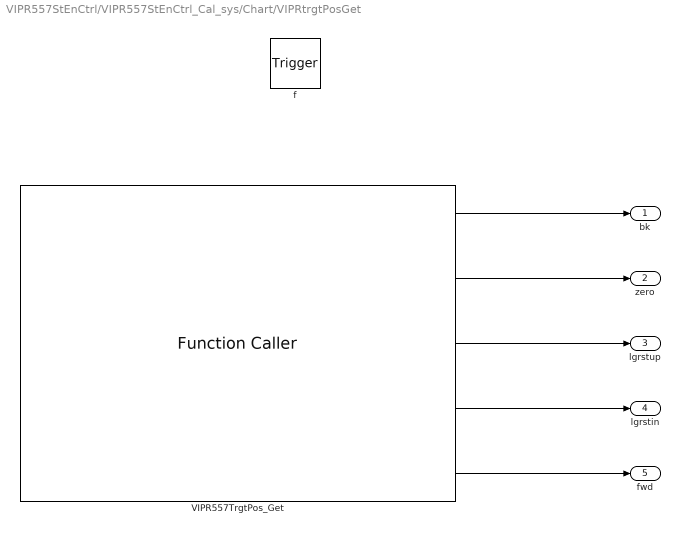
== system VIPR557StEnCtrl/VIPR557StEnCtrl_Cal_sys/Chart/VIPRtrgtPosGet ==
  f : TriggerPort  TriggerType=function-call  VariantControl=(inherit)
      settings: CopyFcn=Stateflow.SLINSF.SimulinkMan.removeBlockPreDeleteFcn  PreDeleteFcn=Stateflow.SLINSF.SimulinkMan.unsafePredeleteFcn
  VIPR557TrgtPos_Get : FunctionCaller  FunctionPrototype=[SecRwLtStBkReclnTrgtPos,SecRwLtStZeroTrgtPos,SecRwLtStLgrstUpwdDnwdTrgtPos,SecRwLtStLgrstInwdOtwdTrgtPos,SecRwLtStFwdBkwdTrgtPos] = VIPR557TrgtPos_Get()  OutputArgumentSpecifications=uint16(1), uint16(1), uint16(1), uint16(1), uint16(1)
  bk : Outport
  zero : Outport  Port=2
  lgrstup : Outport  Port=3
  lgrstin : Outport  Port=4
  fwd : Outport  Port=5
  wires:
  VIPR557TrgtPos_Get/1 -> bk/1
  VIPR557TrgtPos_Get/3 -> lgrstup/1
  VIPR557TrgtPos_Get/2 -> zero/1
  VIPR557TrgtPos_Get/4 -> lgrstin/1
  VIPR557TrgtPos_Get/5 -> fwd/1

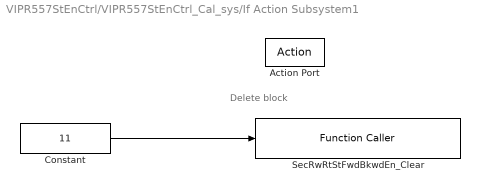
== system VIPR557StEnCtrl/VIPR557StEnCtrl_Cal_sys/If Action Subsystem1 ==
  note: Delete block
  Action Port : ActionPort  ActionType=else
  Constant : Constant  Value=11  OutDataTypeStr=uint8
  SecRwRtStFwdBkwdEn_Clear : FunctionCaller  FunctionPrototype=SecRwRtStFwdBkwdEn_Clear(data)  InputArgumentSpecifications=uint8(1)
  wires:
  Constant/1 -> SecRwRtStFwdBkwdEn_Clear/1

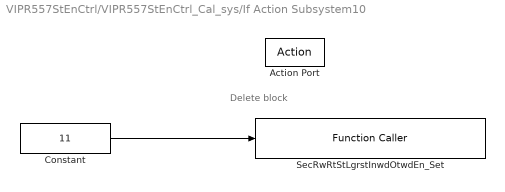
== system VIPR557StEnCtrl/VIPR557StEnCtrl_Cal_sys/If Action Subsystem10 ==
  note: Delete block
  Action Port : ActionPort  ActionType=then
  Constant : Constant  Value=11  OutDataTypeStr=uint8
  SecRwRtStLgrstInwdOtwdEn_Set : FunctionCaller  FunctionPrototype=SecRwRtStLgrstInwdOtwdEn_Set(data)  InputArgumentSpecifications=uint8(1)
  wires:
  Constant/1 -> SecRwRtStLgrstInwdOtwdEn_Set/1

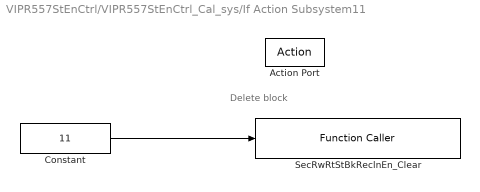
== system VIPR557StEnCtrl/VIPR557StEnCtrl_Cal_sys/If Action Subsystem11 ==
  note: Delete block
  Action Port : ActionPort  ActionType=else
  Constant : Constant  Value=11  OutDataTypeStr=uint8
  SecRwRtStBkReclnEn_Clear : FunctionCaller  FunctionPrototype=SecRwRtStBkReclnEn_Clear(data)  InputArgumentSpecifications=uint8(1)
  wires:
  Constant/1 -> SecRwRtStBkReclnEn_Clear/1

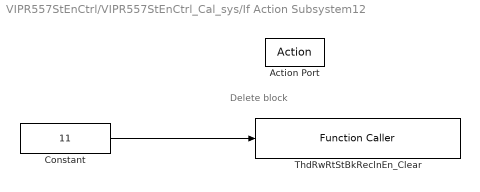
== system VIPR557StEnCtrl/VIPR557StEnCtrl_Cal_sys/If Action Subsystem12 ==
  note: Delete block
  Action Port : ActionPort  ActionType=else
  Constant : Constant  Value=11  OutDataTypeStr=uint8
  ThdRwRtStBkReclnEn_Clear : FunctionCaller  FunctionPrototype=ThdRwRtStBkReclnEn_Clear(data)  InputArgumentSpecifications=uint8(1)
  wires:
  Constant/1 -> ThdRwRtStBkReclnEn_Clear/1

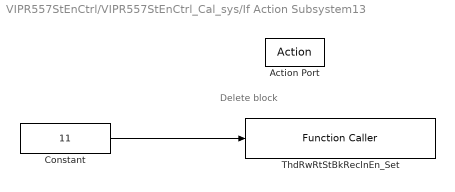
== system VIPR557StEnCtrl/VIPR557StEnCtrl_Cal_sys/If Action Subsystem13 ==
  note: Delete block
  Action Port : ActionPort  ActionType=then
  Constant : Constant  Value=11  OutDataTypeStr=uint8
  ThdRwRtStBkReclnEn_Set : FunctionCaller  FunctionPrototype=ThdRwRtStBkReclnEn_Set(data)  InputArgumentSpecifications=uint8(1)
  wires:
  Constant/1 -> ThdRwRtStBkReclnEn_Set/1

== system VIPR557StEnCtrl/VIPR557StEnCtrl_Cal_sys/If Action Subsystem14 ==
  note: Delete block
  Action Port : ActionPort  ActionType=then
  Constant : Constant  Value=11  OutDataTypeStr=uint8
  SecRwRtStBkReclnEn_Set : FunctionCaller  FunctionPrototype=SecRwRtStBkReclnEn_Set(data)  InputArgumentSpecifications=uint8(1)
  wires:
  Constant/1 -> SecRwRtStBkReclnEn_Set/1

== system VIPR557StEnCtrl/VIPR557StEnCtrl_Cal_sys/If Action Subsystem15 ==
  note: Delete block
  Action Port : ActionPort  ActionType=else
  Constant : Constant  Value=11  OutDataTypeStr=uint8
  ThdRwRtStFwdBkwdEn_Clear : FunctionCaller  FunctionPrototype=ThdRwRtStFwdBkwdEn_Clear(data)  InputArgumentSpecifications=uint8(1)
  wires:
  Constant/1 -> ThdRwRtStFwdBkwdEn_Clear/1

== system VIPR557StEnCtrl/VIPR557StEnCtrl_Cal_sys/If Action Subsystem16 ==
  note: Delete block
  Action Port : ActionPort  ActionType=then
  Constant : Constant  Value=11  OutDataTypeStr=uint8
  ThdRwRtStFwdBkwdEn_Set : FunctionCaller  FunctionPrototype=ThdRwRtStFwdBkwdEn_Set(data)  InputArgumentSpecifications=uint8(1)
  wires:
  Constant/1 -> ThdRwRtStFwdBkwdEn_Set/1

== system VIPR557StEnCtrl/VIPR557StEnCtrl_Cal_sys/If Action Subsystem17 ==
  note: Delete block
  Action Port : ActionPort  ActionType=else
  Constant : Constant  Value=11  OutDataTypeStr=uint8
  PassStBkReclnEn_Clear : FunctionCaller  FunctionPrototype=PassStBkReclnEn_Clear(data)  InputArgumentSpecifications=uint8(1)
  wires:
  Constant/1 -> PassStBkReclnEn_Clear/1

== system VIPR557StEnCtrl/VIPR557StEnCtrl_Cal_sys/If Action Subsystem18 ==
  note: Delete block
  Action Port : ActionPort  ActionType=then
  Constant : Constant  Value=11  OutDataTypeStr=uint8
  PassStBkReclnEn_Set : FunctionCaller  FunctionPrototype=PassStBkReclnEn_Set(data)  InputArgumentSpecifications=uint8(1)
  wires:
  Constant/1 -> PassStBkReclnEn_Set/1

== system VIPR557StEnCtrl/VIPR557StEnCtrl_Cal_sys/If Action Subsystem19 ==
  note: Delete block
  Action Port : ActionPort  ActionType=else
  Constant : Constant  Value=11  OutDataTypeStr=uint8
  PassStFwdBkwdEn_Clear : FunctionCaller  FunctionPrototype=PassStFwdBkwdEn_Clear(data)  InputArgumentSpecifications=uint8(1)
  wires:
  Constant/1 -> PassStFwdBkwdEn_Clear/1

== system VIPR557StEnCtrl/VIPR557StEnCtrl_Cal_sys/If Action Subsystem2 ==
  note: Delete block
  Action Port : ActionPort  ActionType=then
  Constant : Constant  Value=11  OutDataTypeStr=uint8
  SecRwRtStFwdBkwdEn_Set : FunctionCaller  FunctionPrototype=SecRwRtStFwdBkwdEn_Set(data)  InputArgumentSpecifications=uint8(1)
  wires:
  Constant/1 -> SecRwRtStFwdBkwdEn_Set/1

== system VIPR557StEnCtrl/VIPR557StEnCtrl_Cal_sys/If Action Subsystem20 ==
  note: Delete block
  Action Port : ActionPort  ActionType=then
  Constant : Constant  Value=11  OutDataTypeStr=uint8
  PassStFwdBkwdEn_Set : FunctionCaller  FunctionPrototype=PassStFwdBkwdEn_Set(data)  InputArgumentSpecifications=uint8(1)
  wires:
  Constant/1 -> PassStFwdBkwdEn_Set/1

== system VIPR557StEnCtrl/VIPR557StEnCtrl_Cal_sys/If Action Subsystem21 ==
  note: Delete block
  Action Port : ActionPort  ActionType=else
  Constant : Constant  Value=11  OutDataTypeStr=uint8
  ZeroREn_Clear : FunctionCaller  FunctionPrototype=ZeroREn_Clear(data)  InputArgumentSpecifications=uint8(1)
  wires:
  Constant/1 -> ZeroREn_Clear/1

== system VIPR557StEnCtrl/VIPR557StEnCtrl_Cal_sys/If Action Subsystem22 ==
  note: Delete block
  Action Port : ActionPort  ActionType=then
  Constant : Constant  Value=11  OutDataTypeStr=uint8
  ZeroREn_Set : FunctionCaller  FunctionPrototype=ZeroREn_Set(data)  InputArgumentSpecifications=uint8(1)
  wires:
  Constant/1 -> ZeroREn_Set/1

== system VIPR557StEnCtrl/VIPR557StEnCtrl_Cal_sys/If Action Subsystem3 ==
  note: Delete block
  note: Delete block
  note: Delete block
  Action Port : ActionPort  ActionType=else
  Constant : Constant  Value=11  OutDataTypeStr=uint8
  ThdRwLtStBkReclnEn_Clear : FunctionCaller  FunctionPrototype=ThdRwLtStBkReclnEn_Clear(data)  InputArgumentSpecifications=uint8(1)
  wires:
  Constant/1 -> ThdRwLtStBkReclnEn_Clear/1

== system VIPR557StEnCtrl/VIPR557StEnCtrl_Cal_sys/If Action Subsystem4 ==
  note: Delete block
  note: Delete block
  note: Delete block
  Action Port : ActionPort  ActionType=then
  Constant : Constant  Value=11  OutDataTypeStr=uint8
  ThdRwLtStBkReclnEn_Set : FunctionCaller  FunctionPrototype=ThdRwLtStBkReclnEn_Set(data)  InputArgumentSpecifications=uint8(1)
  wires:
  Constant/1 -> ThdRwLtStBkReclnEn_Set/1

== system VIPR557StEnCtrl/VIPR557StEnCtrl_Cal_sys/If Action Subsystem5 ==
  note: Delete block
  note: Delete block
  note: Delete block
  Action Port : ActionPort  ActionType=else
  Constant : Constant  Value=11  OutDataTypeStr=uint8
  ThdRwLtStFwdBkwdEn_Clear : FunctionCaller  FunctionPrototype=ThdRwLtStFwdBkwdEn_Clear(data)  InputArgumentSpecifications=uint8(1)
  wires:
  Constant/1 -> ThdRwLtStFwdBkwdEn_Clear/1

== system VIPR557StEnCtrl/VIPR557StEnCtrl_Cal_sys/If Action Subsystem6 ==
  note: Delete block
  note: Delete block
  note: Delete block
  Action Port : ActionPort  ActionType=then
  Constant : Constant  Value=11  OutDataTypeStr=uint8
  ThdRwLtStFwdBkwdEn_Set : FunctionCaller  FunctionPrototype=ThdRwLtStFwdBkwdEn_Set(data)  InputArgumentSpecifications=uint8(1)
  wires:
  Constant/1 -> ThdRwLtStFwdBkwdEn_Set/1

== system VIPR557StEnCtrl/VIPR557StEnCtrl_Cal_sys/If Action Subsystem7 ==
  note: Delete block
  Action Port : ActionPort  ActionType=else
  Constant : Constant  Value=11  OutDataTypeStr=uint8
  SecRwRtStLgrstUpwdDnwdEn_Clear : FunctionCaller  FunctionPrototype=SecRwRtStLgrstUpwdDnwdEn_Clear(data)  InputArgumentSpecifications=uint8(1)
  wires:
  Constant/1 -> SecRwRtStLgrstUpwdDnwdEn_Clear/1

== system VIPR557StEnCtrl/VIPR557StEnCtrl_Cal_sys/If Action Subsystem8 ==
  note: Delete block
  Action Port : ActionPort  ActionType=then
  Constant : Constant  Value=11  OutDataTypeStr=uint8
  SecRwRtStLgrstUpwdDnwdEn_Set : FunctionCaller  FunctionPrototype=SecRwRtStLgrstUpwdDnwdEn_Set(data)  InputArgumentSpecifications=uint8(1)
  wires:
  Constant/1 -> SecRwRtStLgrstUpwdDnwdEn_Set/1

== system VIPR557StEnCtrl/VIPR557StEnCtrl_Cal_sys/If Action Subsystem9 ==
  note: Delete block
  Action Port : ActionPort  ActionType=else
  Constant : Constant  Value=11  OutDataTypeStr=uint8
  SecRwRtStLgrstInwdOtwdEn_Clear : FunctionCaller  FunctionPrototype=SecRwRtStLgrstInwdOtwdEn_Clear(data)  InputArgumentSpecifications=uint8(1)
  wires:
  Constant/1 -> SecRwRtStLgrstInwdOtwdEn_Clear/1

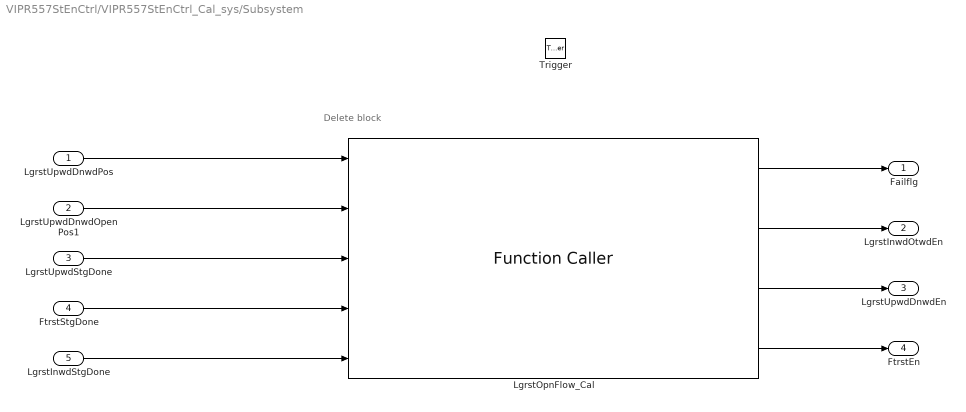
== system VIPR557StEnCtrl/VIPR557StEnCtrl_Cal_sys/Subsystem ==
  note: Delete block
  LgrstUpwdDnwdPos : Inport
  LgrstUpwdDnwdOpenPos1 : Inport  Port=2
  LgrstUpwdStgDone : Inport  Port=3
  FtrstStgDone : Inport  Port=4
  LgrstInwdStgDone : Inport  Port=5
  Trigger : TriggerPort  TriggerType=function-call  VariantControl=Variant  PortDimensions=1
  LgrstOpnFlow_Cal : FunctionCaller  FunctionPrototype=[Failflg,LgrstInwdOtwdEn,LgrstUpwdDnwdEn,FtrstEn] = LgrstOpnFlow_Cal(LgrstUpwdDnwdPos,LgrstUpwdDnwdOpenPos1,LgrstUpwdStgDone,FtrstStgDone,LgrstInwdStgDone)  InputArgumentSpecifications=uint16(1), uint16(1), boolean(true), boolean(true), boolean(true)  OutputArgumentSpecifications=boolean(true), boolean(true), boolean(true), boolean(true)
  Failflg : Outport
  LgrstInwdOtwdEn : Outport  Port=2
  LgrstUpwdDnwdEn : Outport  Port=3
  FtrstEn : Outport  Port=4
  wires:
  LgrstOpnFlow_Cal/2 -> LgrstInwdOtwdEn/1
  LgrstUpwdDnwdPos/1 -> LgrstOpnFlow_Cal/1
  LgrstOpnFlow_Cal/3 -> LgrstUpwdDnwdEn/1
  FtrstStgDone/1 -> LgrstOpnFlow_Cal/4
  LgrstUpwdStgDone/1 -> LgrstOpnFlow_Cal/3
  LgrstOpnFlow_Cal/4 -> FtrstEn/1
  LgrstInwdStgDone/1 -> LgrstOpnFlow_Cal/5
  LgrstUpwdDnwdOpenPos1/1 -> LgrstOpnFlow_Cal/2
  LgrstOpnFlow_Cal/1 -> Failflg/1

== stateflow chart VIPR557StEnCtrl/VIPR557StEnCtrl_Cal_sys/Chart ==
  state PosAvlOut=VIPRTrgtPosChk [function]
  state [bk,zero,lgrstup,lgrstin,fwd]=VIPRtrgtPosGet [function]
  state FwdBkwd [function]
    (default) -> (junction 279)
    (junction 279) -> (junction 280) [order 1] : [PassStFwdBkwdStgDone]
    (junction 279) -> (junction 282) [order 2] : {PassStFwdBkwdEn=1;}
    (junction 280) -> (junction 281)
    (junction 281) -> (junction 282)
    (junction 282) -> (junction 283)
  (default) -> (junction 205) : {
      | ThdRwLtStBkReclnEn = 0;
      | SecRwLtStBkReclnEn = 0;
      | SecRwLtStFrwdBkwdEn = 0;
      | SecRwLtStLgrstOtwdInwdEn = 0;
      | SecRwLtStLgrstUpwdDnwdEn = 0;
      | ThdRwLtStFwdBkwdEn = 0;
      | ThdRwRtStBkReclnEn = 0;
      | ThdRwRtStFwdBkwdEn = 0;
      | PassStBkReclnEn = 0;
      | PassStFwdBkwdEn = 0;
      | SecRwStZeroEn = 0;
      | }
  (junction 205) -> (junction 207) [order 1] : [FirstTrig]
  (junction 205) -> (junction 211) [order 2]
  (junction 207) -> (junction 209) : {PosAvl=0;}
  (junction 209) -> (junction 211)
  (junction 211) -> (junction 1)
  (junction 1) -> (junction 22) [order 1] : [(!is7s)||ThdRwLtStBkReclnStgDone]
  (junction 1) -> (junction 26) [order 2] : {ThdRwLtStBkReclnEn = 1;}
  (junction 22) -> (junction 24)
  (junction 24) -> (junction 26)
  (junction 26) -> (junction 29)
  (junction 29) -> (junction 31) [order 1] : [(!is7s)||ThdRwLtStFwdBkwdStgDone]
  (junction 29) -> (junction 35) [order 2] : {
      | ThdRwLtStFwdBkwdEn = 1;
      | }
  (junction 31) -> (junction 33)
  (junction 33) -> (junction 35)
  (junction 35) -> (junction 105)
  (junction 105) -> (junction 109) [order 1] : [ThdRwRtStBkReclnStgDone]
  (junction 105) -> (junction 106) [order 2] : {ThdRwRtStBkReclnEn = 1;}
  (junction 109) -> (junction 110)
  (junction 110) -> (junction 106)
  (junction 106) -> (junction 108)
  (junction 108) -> (junction 117) [order 1] : [ThdRwRtStFwdBkwdStgDone]
  (junction 108) -> (junction 107) [order 2] : {
      | ThdRwRtStFwdBkwdEn = 1;
      | }
  (junction 117) -> (junction 114)
  (junction 114) -> (junction 107)
  (junction 107) -> (junction 248)
  (junction 248) -> (junction 253) [order 1] : [NotMovPassStFlg]
  (junction 248) -> (junction 249) [order 2]
  (junction 253) -> (junction 243)
  (junction 249) -> (junction 245) [order 1] : [ NotMovPassStBkReclnFlg]
  (junction 249) -> (junction 247) [order 2]
  (junction 245) -> (junction 242) : {FwdBkwd();}
  (junction 247) -> (junction 236) [order 1] : [HalfMovPassStBkReclnFlg||IfVeSMSuPassStBkReclnUpwdDnwdPosV==1]
  (junction 247) -> (junction 237) [order 2]
  (junction 236) -> (junction 240)
  (junction 237) -> (junction 241) [order 1] : [PassStBkReclnStgDone]
  (junction 237) -> (junction 246) [order 2] : {PassStBkReclnEn=1;}
  (junction 241) -> (junction 244)
  (junction 244) -> (junction 246)
  (junction 246) -> (junction 292)
  (junction 292) -> (junction 298)
  (junction 298) -> (junction 250)
  (junction 250) -> (junction 251) [order 1] : [!PassStCshnFldFailflg&&!PassStFwdBkwdStgDone]
  (junction 250) -> (junction 238) [order 2]
  (junction 251) -> (junction 239) : {PassStFwdBkwdEn=1;}
  (junction 239) -> (junction 238)
  (junction 238) -> (junction 252)
  (junction 240) -> (junction 252)
  (junction 242) -> (junction 240)
  (junction 243) -> (junction 242)
  (junction 252) -> (junction 153)
  (junction 153) -> (junction 157) [order 1] : [Stg1Done]
  (junction 157) -> (junction 216) [order 1] : [!PosAvl]
  (junction 153) -> (junction 166) [order 2]
  (junction 157) -> (junction 220) [order 2]
  (junction 216) -> (junction 218) : {PosAvl = VIPRTrgtPosChk ();}
  (junction 218) -> (junction 220)
  (junction 220) -> (junction 159)
  (junction 159) -> (junction 38) [order 1] : [PosAvl]
  (junction 159) -> (junction 169) [order 2]
  (junction 38) -> (junction 196) : {[bktrgt,zerotrgt,lgrstuptrgt,lgrstintrgt,fwdtrgt]=VIPRtrgtPosGet();}
  (junction 196) -> (junction 40) [order 1] : [IfVeSMSuSecRwLtStBkReclnUpwdDnwdPos>bktrgt&&!SecRwLtStBkReclnStgDone]
  (junction 196) -> (junction 44) [order 2]
  (junction 40) -> (junction 42) : {SecRwLtStBkReclnEn = 1;}
  (junction 42) -> (junction 44)
  (junction 44) -> (junction 47)
  (junction 47) -> (junction 49) [order 1] : [IfVeSMSuSecRwLtStLgrstOtwdInwdPos >lgrstintrgt &&!SecRwLtStLgrstOtwdInwdStgDone]
  (junction 47) -> (junction 53) [order 2]
  (junction 49) -> (junction 51) : {SecRwLtStLgrstOtwdInwdEn = 1;}
  (junction 51) -> (junction 53)
  (junction 53) -> (junction 56)
  (junction 56) -> (junction 58) [order 1] : [IfVeSMSuSecRwLtStLgrstUpwdDnwdPos >lgrstuptrgt && !SecRwLtStLgrstUpwdDnwdStgDone]
  (junction 56) -> (junction 62) [order 2]
  (junction 58) -> (junction 60) : {SecRwLtStLgrstUpwdDnwdEn = 1;}
  (junction 60) -> (junction 62)
  (junction 62) -> (junction 172)
  (junction 172) -> (junction 174) [order 1] : [IfVeSMSuSecRwRtStZeroPos >zerotrgt && !ZeroRStgDone]
  (junction 172) -> (junction 178) [order 2]
  (junction 174) -> (junction 176) : {SecRwStZeroEn = 1; }
  (junction 176) -> (junction 178)
  (junction 178) -> (junction 65)
  (junction 65) -> (junction 67) [order 1] : [
      | (IfVeSMSuSecRwLtStBkReclnUpwdDnwdPos<=bktrgt||SecRwLtStBkReclnStgDone)&&...
      | (IfVeSMSuSecRwLtStLgrstOtwdInwdPos <=lgrstintrgt ||SecRwLtStLgrstOtwdInwdStgDone) &&...
      | (IfVeSMSuSecRwLtStLgrstUpwdDnwdPos <=lgrstuptrgt ||SecRwLtStLgrstUpwdDnwdStgDone)&&...
      | (IfVeSMSuSecRwRtStZeroPos <=zerotrgt || ZeroRStgDone)
      | ]
  (junction 67) -> (junction 69) [order 1] : [SecRwLtStFrwdBkwdStgDone]
  (junction 69) -> (junction 76) [order 1] : [SecRwLtStBkReclnStgDone]
  (junction 65) -> (junction 87) [order 2]
  (junction 67) -> (junction 73) [order 2] : {SecRwLtStFrwdBkwdEn =1;}
  (junction 69) -> (junction 71) [order 2] : {SecRwLtStBkReclnEn = 1;}
  (junction 76) -> (junction 78)
  (junction 78) -> (junction 71)
  (junction 71) -> (junction 181)
  (junction 181) -> (junction 183) [order 1] : [ZeroRStgDone]
  (junction 181) -> (junction 187) [order 2] : {SecRwStZeroEn = 1; }
  (junction 183) -> (junction 185)
  (junction 185) -> (junction 187)
  (junction 187) -> (junction 81) : {LgrstOpn;}
  (junction 169) -> (junction 166)
  (junction 87) -> (junction 169)
  (junction 73) -> (junction 87)
  (junction 81) -> (junction 73)
  data: PosAvlOut function_output; bk function_output; zero function_output; lgrstup function_output; lgrstin function_output; fwd function_output; HalfMovPassStBkReclnFlg input; IfVeSMSuSecRwLtStBkReclnUpwdDnwdPos input; IfVeSMSuSecRwLtStLgrstOtwdInwdPos input; IfVeSMSuSecRwLtStLgrstUpwdDnwdPos input; SecRwLtStBkReclnStgDone input; SecRwLtStFrwdBkwdStgDone input; SecRwLtStLgrstOtwdInwdStgDone input; SecRwLtStLgrstUpwdDnwdStgDone input; ThdRwLtStBkReclnStgDone input; ThdRwLtStFwdBkwdStgDone input; VIPLR2LBkReclnUpwdDnwdTrgtPos input; VIPLR2LFwdBkwdTrgtPos input; VIPLR2LLgrstInwdOtwdTrgtPos input; VIPLR2LLgrstUpwdDnwdTrgtPos input; SecRwLtStBkReclnEn output boolean; SecRwLtStFrwdBkwdEn output boolean; SecRwLtStLgrstOtwdInwdEn output boolean; ThdRwLtStBkReclnEn output boolean; ThdRwLtStFwdBkwdEn output boolean; SecRwLtStLgrstUpwdDnwdEn output boolean; ThdRwRtStBkReclnEn output boolean; ThdRwRtStFwdBkwdEn output boolean; PassStBkReclnEn output boolean; PassStFwdBkwdEn output boolean; ThdRwRtStBkReclnStgDone input; ThdRwRtStFwdBkwdStgDone input; PassStBkReclnStgDone input; PassStFwdBkwdStgDone input; NotMovPassStFlg input boolean; NotMovPassStBkReclnFlg input boolean; IfVeSMSuSecRwRtStZeroPos input; VIPRMdR2RZeroTrgtPos input; ZeroRStgDone input boolean; Stg1Done input boolean; SecRwStZeroEn output boolean; PosAvl output boolean; bktrgt local uint16; zerotrgt local uint16; lgrstuptrgt local uint16; lgrstintrgt local uint16; fwdtrgt local uint16; FirstTrig input boolean; is7s input; IfVeSMSuPassStBkReclnUpwdDnwdPosV input; PassStCshnFldFailflg input boolean
  events: LgrstOpn output FUNCTION_CALL_EVENT
